simulink model "PwrLimit"  (R2019b)
settings: Solver=VariableStepAuto  StartTime=0.0  StopTime=10.0  RelTol=1e-3
libraries: simulink x1
settings Model: Creator=YJR  LastModifiedBy=YJR

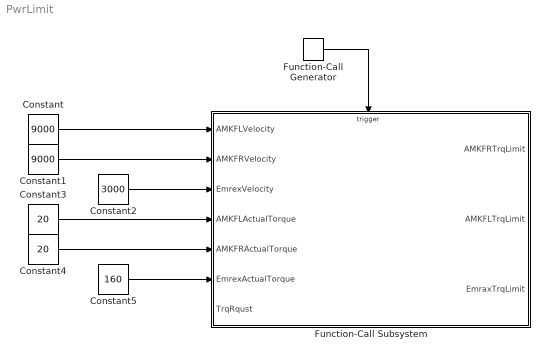
== system PwrLimit ==
  Constant : Constant  Value=9000
  Constant1 : Constant  Value=9000
  Constant2 : Constant  Value=3000
  Constant3 : Constant  Value=20
  Constant4 : Constant  Value=20
  Constant5 : Constant  Value=160
  Function-Call Generator : simulink/Ports & Subsystems/Function-Call Generator  sample_time=0.01  numberOfIterations=1
  Function-Call Subsystem : Subsystem  TreatAsAtomicUnit=on
  wires:
  Function-Call Generator/1 -> Function-Call Subsystem/Trigger
  Constant/1 -> Function-Call Subsystem/1(AMKFLVelocity)
  Constant1/1 -> Function-Call Subsystem/2(AMKFRVelocity)
  Constant3/1 -> Function-Call Subsystem/4(AMKFLActualTorque)
  Constant4/1 -> Function-Call Subsystem/5(AMKFRActualTorque)
  Constant5/1 -> Function-Call Subsystem/6(EmrexActualTorque)
  Constant2/1 -> Function-Call Subsystem/3(EmrexVelocity)

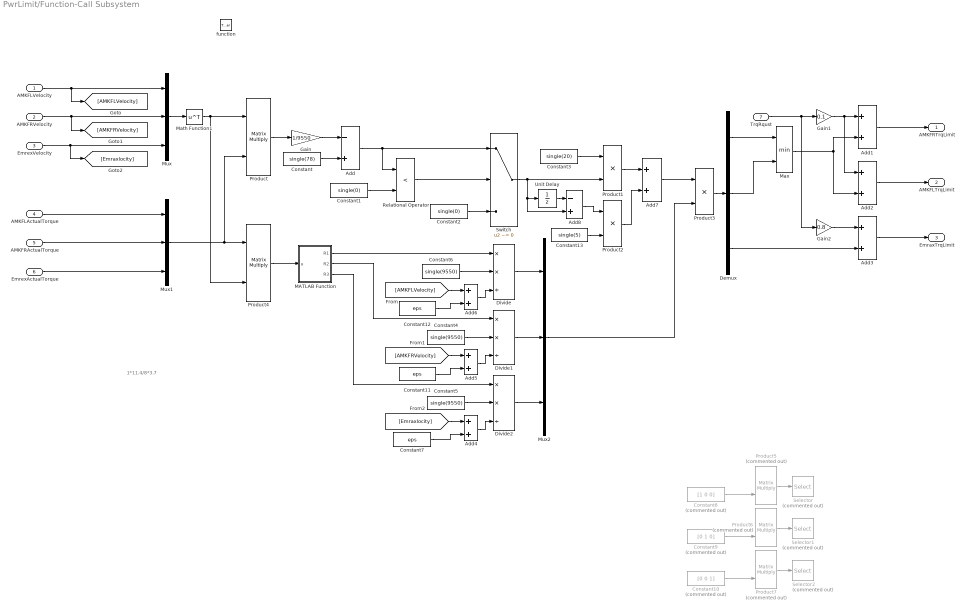
== system PwrLimit/Function-Call Subsystem ==
  note: 1*11.4/8*3.7
  AMKFLVelocity : Inport
  AMKFRVelocity : Inport  Port=2
  EmrexVelocity : Inport  Port=3
  AMKFLActualTorque : Inport  Port=4
  AMKFRActualTorque : Inport  Port=5
  EmrexActualTorque : Inport  Port=6
  TrqRqust : Inport  Port=7
  function : TriggerPort  TriggerType=function-call  VariantControl=Variant
  Add : Sum  Inputs=-+
  Add{1..7} (7 alike) : Sum
  Add8 : Sum  Inputs=-+
  Constant : Constant  Value=single(78)
  Constant1 : Constant  Value=single(0)
  Constant10 : Constant  Commented=on  Value=[0 0 1]
  Constant11 : Constant  Value=eps
  Constant12 : Constant  Value=eps
  Constant13 : Constant  Value=single(5)
  Constant2 : Constant  Value=single(0)
  Constant3 : Constant  Value=single(20)
  Constant4 : Constant  Value=single(9550)
  Constant5 : Constant  Value=single(9550)
  Constant6 : Constant  Value=single(9550)
  Constant7 : Constant  Value=eps
  Constant8 : Constant  Commented=on  Value=[1 0 0]
  Constant9 : Constant  Commented=on  Value=[0 1 0]
  Demux : Demux  Outputs=3
  Divide : Product  Inputs=**/
  Divide1 : Product  Inputs=**/
  Divide2 : Product  Inputs=**/
  Gain : Gain  Gain=1/9550
  Gain1 : Gain  Gain=0.1
  Gain2 : Gain  Gain=0.8
  MATLAB Function : MATLAB Function  TreatAsAtomicUnit=on
  Math Function1 : Math  Operator=transpose  SignedPower=off  SaturateOnIntegerOverflow=on
  Max : MinMax  Inputs=2
  Mux : Mux  Inputs=3
  Mux1 : Mux  Inputs=3
  Mux2 : Mux  Inputs=3
  Product : Product  Multiplication=Matrix(*)
  Product1 : Product
  Product2 : Product
  Product3 : Product
  Product4 : Product  Multiplication=Matrix(*)
  Product5 : Product  Commented=on  Multiplication=Matrix(*)
  Product6 : Product  Commented=on  Multiplication=Matrix(*)
  Product7 : Product  Commented=on  Multiplication=Matrix(*)
  Relational Operator : RelationalOperator  Operator=<  OutDataTypeStr=boolean  RndMeth=Simplest
  Selector : Selector  Commented=on  InputPortWidth=3  IndexOptions=Index vector (dialog)  Indices=1  OutputSizes=1
  Selector1 : Selector  Commented=on  InputPortWidth=3  IndexOptions=Index vector (dialog)  Indices=2  OutputSizes=1
  Selector2 : Selector  Commented=on  InputPortWidth=3  IndexOptions=Index vector (dialog)  Indices=3  OutputSizes=1
  Switch : Switch  Criteria=u2 ~= 0
  Unit Delay : UnitDelay  SampleTime=-1  HasFrameUpgradeWarning=on
  AMKFRTrqLimit : Outport
  AMKFLTrqLimit : Outport  Port=2
  EmraxTrqLimit : Outport  Port=3
  wires:
  AMKFRVelocity/1 -> [AMKFRVelocity], Mux/2
  EmrexVelocity/1 -> [Emraxlocity], Mux/3
  AMKFLVelocity/1 -> Mux/1, [AMKFLVelocity]
  AMKFLActualTorque/1 -> Mux1/1
  AMKFRActualTorque/1 -> Mux1/2
  EmrexActualTorque/1 -> Mux1/3
  Mux/1 -> Math Function1/1
  Mux1/1 -> Product4/1, Product/2
  Product/1 -> Gain/1
  Math Function1/1 -> Product4/2, Product/1
  Gain/1 -> Add/1
  Constant/1 -> Add/2
  Add/1 -> Switch/1, Relational Operator/1
  Constant1/1 -> Relational Operator/2
  Relational Operator/1 -> Switch/2
  Constant2/1 -> Switch/3
  Switch/1 -> Product1/2, Add8/2, Unit Delay/1
  Constant3/1 -> Product1/1
  Add7/1 -> Product3/1
  TrqRqust/1 -> Gain1/1, Gain2/1
  Gain1/1 -> Add2/1, Add1/1
  Constant6/1 -> Divide/2
  Gain2/1 -> Add3/1
  Add1/1 -> AMKFRTrqLimit/1
  Add2/1 -> AMKFLTrqLimit/1
  Add3/1 -> EmraxTrqLimit/1
  Product4/1 -> MATLAB Function/1(u)
  Constant8/1 -> Product5/2
  Product5/1 -> Selector/1
  Constant9/1 -> Product6/2
  Constant10/1 -> Product7/2
  Product6/1 -> Selector1/1
  Product7/1 -> Selector2/1
  MATLAB Function/1(R1) -> Divide/1
  [AMKFLVelocity] -> Add6/1
  [AMKFRVelocity] -> Add5/1
  MATLAB Function/2(R2) -> Divide1/1
  Constant4/1 -> Divide1/2
  Constant5/1 -> Divide2/2
  MATLAB Function/3(R3) -> Divide2/1
  [Emraxlocity] -> Add4/1
  Divide/1 -> Mux2/1
  Divide1/1 -> Mux2/2
  Divide2/1 -> Mux2/3
  Mux2/1 -> Product3/2
  Add4/1 -> Divide2/3
  Constant7/1 -> Add4/2
  Add5/1 -> Divide1/3
  Constant11/1 -> Add5/2
  Add6/1 -> Divide/3
  Constant12/1 -> Add6/2
  Demux/1 -> Max/1
  Demux/2 -> Max/2
  Demux/3 -> Add3/2
  Max/1 -> Add1/2, Add2/2
  Constant13/1 -> Product2/2
  Product2/1 -> Add7/2
  Product1/1 -> Add7/1
  Unit Delay/1 -> Add8/1
  Add8/1 -> Product2/1
  Product3/1 -> Demux/1

== matlab function PwrLimit/Function-Call Subsystem/MATLAB Function ==
  data: u input; R1 output; R2 output; R3 output
function [R1,R2,R3] = fcn(u)

y1 = u(1,1);
y2 = u(2,2);
y3 = u(3,3);
R1 = y1/(y1+y2+y3);
R2 = y2/(y1+y2+y3);
R3 = y3/(y1+y2+y3);
